simulink library "lib_dGrid"  (R2023b)
settings: Solver=VariableStepAuto  StartTime=0.0  StopTime=10.0  RelTol=1e-3
values from neighbouring files (symbols this model uses):
  C_PM = 10e-3    (= 0.01)    [my_MMC_param.m]
  Cbase = 1/Zbase/wb    (= 3.10849498226e-05)    [my_MMC_param.m]
  f0 = 50/fb    (= 1)    [my_MMC_param.m]
  Fn_filter = 1000    [my_MMC_param.m]
  Fnom = 50    [my_MMC_param.m]
  GFL_APC = 1    [Analysis_Main.m]    (also in initSimu.m; my_MMC_param.m)
  GFL_DVC = 2    [Analysis_Main.m]    (also in initSimu.m; my_MMC_param.m)
  GFM_APC = 3; (values programmed in EMT models)    [Analysis_Main.m]    (also in initSimu.m; my_MMC_param.m = 3)
  GFM_VF = 0    [my_MMC_param.m]
  Ibase = 2*Sbase/(3*Ubase)    [my_MMC_param.m]
  Idcb = Sbase/Udcb    [my_MMC_param.m]
  Ki_Iccsc = 5.15    [my_MMC_param.m]
  Ki_Ireg = CCCTRL.CC.ki    [my_MMC_param.m]
  Ki_Izscc = 100    [my_MMC_param.m]
  Ki_PLL = 1/(CCCTRL.PLL.v0*CCCTRL.PLL.T^2)    [my_MMC_param.m]
  Ki_Preg = 1.0*10    (= 10)    [my_MMC_param.m]
  Ki_Qreg = 1.0*10    (= 10)    [my_MMC_param.m]
  Ki_VAC_GFL = 50    [my_MMC_param.m]
  Ki_VACreg = 10    [my_MMC_param.m]
  Ki_VDCreg = 10    [my_MMC_param.m]
  Ki_WtReg = Kp_WtReg / 0.025    (= 1600)    [my_MMC_param.m]
  Kp_Iccsc = 0.21    [my_MMC_param.m]
  Kp_Ireg = CCCTRL.CC.kp    [my_MMC_param.m]
  Kp_Izscc = 10    [my_MMC_param.m]
  Kp_PLL = 2/CCCTRL.PLL.v0/CCCTRL.PLL.T    [my_MMC_param.m]
  Kp_Preg = 0.5/3*1    (= 0.166666666667)    [my_MMC_param.m]
  Kp_Qreg = 0.5/3*1    (= 0.166666666667)    [my_MMC_param.m]
  Kp_VAC_GFL = 0.5    [my_MMC_param.m]
  Kp_VACreg = 0.01    [my_MMC_param.m]
  Kp_VDCreg = 1    [my_MMC_param.m]
  Kp_WtReg = 40    [my_MMC_param.m]
  Kpv_GFM = 1    [my_MMC_param.m]
  Kpwm = 0.5    [my_MMC_param.m]
  Larm = Larm_pu*(Zbase/wb)    (= 0.0488923985178)    [my_MMC_param.m]
  Lff = Larm_pu/2    (= 0.075)    [my_MMC_param.m]
  Limits_Ireg = [ 2.0  -2.0]    [my_MMC_param.m]
  Limits_Preg = [ 2, -2 ]    [my_MMC_param.m]
  Limits_Qreg = 2*[ 0.42, -0.42 ]    [my_MMC_param.m]
  Limits_VACreg = [ 1.3  -1.3]    [my_MMC_param.m]
  Limits_VDCreg = [ 2.0  -2.0]    [my_MMC_param.m]
  MMC1 = MMC    [Analysis_Main.m]    (also in initSimu.m)
  Nb_PM = 400    [my_MMC_param.m]
  PhaseDelay = 1.0*Ts_Control*2*pi*50    (= 0.0628318530718)    [my_MMC_param.m]
  Pnom = 1000e6    (= 1000000000)    [my_MMC_param.m]
  Rarm = Rarm_pu*Zbase    (= 0.1536)    [my_MMC_param.m]
  Slope_Pref = 0.5    [my_MMC_param.m]
  Slope_Qref = 0.5    [my_MMC_param.m]
  Slope_Vdc_ref = Vnom_dc/2    (= 320000)    [my_MMC_param.m]
  Tdeblock = 1.5    [my_MMC_param.m]
  Ton_CROSSreg = Ton_PQreg+3    (= 7)    [my_MMC_param.m]
  Ton_PQreg = 4    [my_MMC_param.m]
  Ton_VDCreg = 1.5    [my_MMC_param.m]
  Ts = Ts_Control    (= 0.0002)    [my_MMC_param.m]
  Ts_Control = Ts_Power*2    (= 0.0002)    [my_MMC_param.m]
  Ts_Power = 20e-6 * 5    (= 0.0001)    [my_MMC_param.m]
  Ubase = sqrt(2/3)*Vnom_sec    [my_MMC_param.m]
  Udcb = 2*Ubase    [my_MMC_param.m]
  Vc0_PM = 0    [my_MMC_param.m]
  Vnom_dc = 640e3    (= 640000)    [my_MMC_param.m]
  Vnom_sec = 320e3    (= 320000)    [my_MMC_param.m]
  wb = 2*pi*fb    (= 314.159265359)    [my_MMC_param.m]
  Wt_ref_pu = 0.5 * C_PM * (Vnom_dc/Nb_PM)^2 * Nb_PM * 6 / Pnom    (= 0.03072)    [my_MMC_param.m]
undefined symbols (not defined in the file or in its folder): ControlSampleTime, DiscIntNeverNeededParam, MMC, PLL, VSM
libraries: simulink x50, spsCurrentMeasurementLib x20, spsSecondOrderFilterLib x20, spsDiodeLib x12, spsControlledVoltageSourceLib x12, spsSeriesRLCBranchLib x10, spsFirstOrderFilterLib x9, spsVoltageMeasurementLib x8, spsMeanLib x7, FriedrichLibrary x6, $bdroot x6, powerlib_extras x4
(part 1 of 8)
settings Model: Creator=uk081705  LastModifiedBy=uk081705

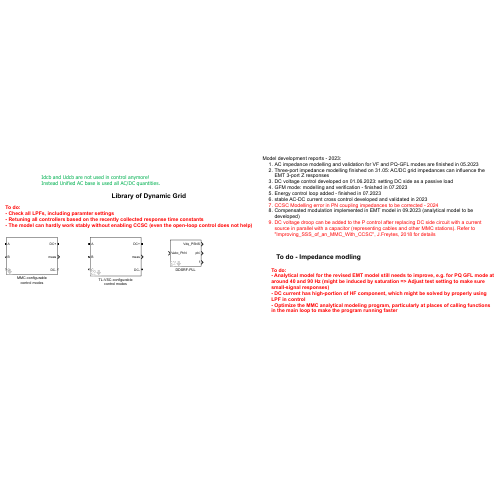
[thumbnail: Simulink's stored preview of the top-level diagram]
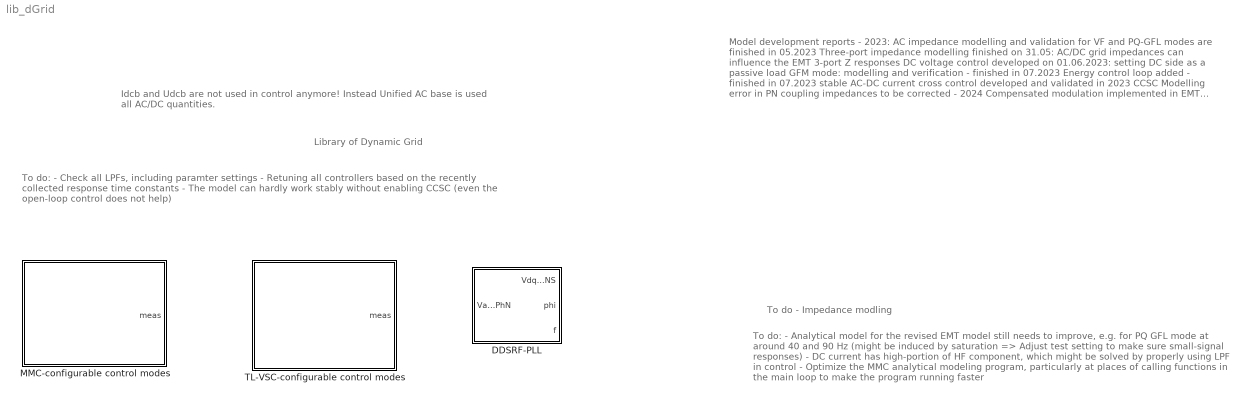
== system lib_dGrid ==
  note: To do:
      | - Check all LPFs, including paramter settings
      | - Retuning all controllers based on the recently collected response time constants
      | - The model can hardly work stably without enabling CCSC (even the open-loop control does not help)
  note: Library of Dynamic Grid
  note: Model development reports - 2023:
      | AC impedance modelling and validation for VF and PQ-GFL modes are finished in 05.2023
      | Three-port impedance modelling finished on 31.05: AC/DC grid impedances can influence the EMT 3-port Z responses
      | DC voltage control developed on 01.06.2023: setting DC side as a passive load
      | GFM mode: modelling and verification - finished in 07.2023
      | Energy control loop added - finished in 07.2023
      | stable AC-DC current cross control developed and validated in 2023
      | CCSC Modelling error in PN coupling impedances to be corrected - 2024
      | Compensated modulation implemented in EMT model in 09.2023 (analytical model to be developed)
      | DC voltage droop can be added to the P control after replacing DC side circuit with a current source in parallel with a capacitor (representing cables and other MMC stations). Refer to "Improving_SSS_of_an_MMC_With_CCSC", J.Freytes, 2018 for details
  note: Idcb and Udcb are not used in control anymore!
      | Instead Unified AC base is used all AC/DC quantities.
  note: To do:
      | - Analytical model for the revised EMT model still needs to improve, e.g. for PQ GFL mode at around 40 and 90 Hz (might be induced by saturation => Adjust test setting to make sure small-signal responses)
      | - DC current has high-portion of HF component, which might be solved by properly using LPF in control
      | - Optimize the MMC analytical modeling program, particularly at places of calling functions in the main loop to make the program running faster
  note: To do - Impedance modling
  DDSRF-PLL : Subsystem  AncestorBlock=FriedrichLibrary/Discrete Stuff/DDSRF-PLL  mask{Kp_PLL=PLL.kp, Ki_PLL=PLL.ki, Kd_PLL=0, Tpt1=0.005, Ts=ControlSampleTime}
      mask prompts: Kp_PLL "Proportional Gain PLL"; Ki_PLL "Integral Gain PLL"; Kd_PLL "Differential Gain PLL"; Tpt1 "PT1 Settling Time"; Ts "SampleTime"
      mask DialogControl DescGroupVar Prompt: DDSRF PLL
      mask DialogControl DescTextVar Prompt: Discrete implementation of a double decoupled sychronous reference frame phase locked loop.
  MMC-configurable control modes : Subsystem  mask{CtrlMode=MMC.CtrlMode, Ctrl=MMC.Ctrl, Set=MMC.Set}
      mask prompts: CtrlMode "GFM-VF0,GFL-APC1,GFL-DVC2, GFM-APC3"; Ctrl "CtrlStru"; Set "SetStru"
      settings: PortSchema="{\"entries\":[{\"content\":{\"sides\":[{\"content\":{\"connectorIds\":[\"LConn1\",\"LConn2\",\"LConn3\"]},\"type\":\"ConnectorPlacement.EquallySpacedRectSide\",\"uuid\":\"c923a6b0-d2fc-4b8e-a4b1-de94c3223959\"},{\"content\":{\"connectorIds\":[\"RConn1\",\"Out1\",\"RConn2\"],\"side\":\"RIGHT\"},\"type\":\"ConnectorPlacement.EquallySpacedRectSide\",\"uuid\":\"6efd3e4a-f3ae-490c-a9d1-2120854778d7\"},{\"content\":{\"side\":\"TOP\"},\"type\":\"ConnectorPlacement.EquallySpacedRectSide\",\"uuid\":\"54cc3c02-aa24-440c-8051-39c65b165fe4\"}]},\"type\":\"ConnectorPlacement.EquallySpacedConnector\",\"uuid\":\"58f4ddb9-74a8-4d52-977f-61a3e301d753\"}],\"packageUris\":[\"http://schema.mathworks.com/mf0/Connector/R2020b\"],\"version\":\"1.0\"}"
      mask DialogControl AAM Prompt: MMC-Averaged Arm Model
  TL-VSC-configurable control modes : Subsystem  AncestorBlock=Library_dynaGrid/MMC - configurable control & operating modes  mask{CtrlMode=MMC1.CtrlMode, Ctrl=MMC1.Ctrl, Set=MMC1.Set}
      mask prompts: CtrlMode "GFM-VF0,GFL-APC1,GFL-DVC2, GFM-APC3"; Ctrl "CtrlStru"; Set "SetStru"
      settings: PortSchema="{\"entries\":[{\"content\":{\"sides\":[{\"content\":{\"connectorIds\":[\"LConn1\",\"LConn2\",\"LConn3\"]},\"type\":\"ConnectorPlacement.EquallySpacedRectSide\",\"uuid\":\"c923a6b0-d2fc-4b8e-a4b1-de94c3223959\"},{\"content\":{\"connectorIds\":[\"RConn1\",\"Out1\",\"RConn2\"],\"side\":\"RIGHT\"},\"type\":\"ConnectorPlacement.EquallySpacedRectSide\",\"uuid\":\"6efd3e4a-f3ae-490c-a9d1-2120854778d7\"},{\"content\":{\"side\":\"TOP\"},\"type\":\"ConnectorPlacement.EquallySpacedRectSide\",\"uuid\":\"54cc3c02-aa24-440c-8051-39c65b165fe4\"}]},\"type\":\"ConnectorPlacement.EquallySpacedConnector\",\"uuid\":\"58f4ddb9-74a8-4d52-977f-61a3e301d753\"}],\"packageUris\":[\"http://schema.mathworks.com/mf0/Connector/R2020b\"],\"version\":\"1.0\"}"
      mask DialogControl AAM Prompt: MMC-Averaged Arm Model

== system lib_dGrid/DDSRF-PLL ==
  Vabc_PhN : Inport
  Angle Integrator [SI] : FriedrichLibrary/Discrete Stuff/Angle Integrator [SI]  Ts=Ts
  Bus Creator : BusCreator  Inputs=2
  Demux1 : Demux  Outputs=2
  PhN->ab0 : FriedrichLibrary/Transformations/PhN->ab0  SystemSampleTime=-1  VariantActivationTime=update diagram  AllowFlexibleInterface=on  Latency=0  AutoFrameSizeCalculation=off
  Selector : Selector  InputPortWidth=3  IndexOptions=Index vector (dialog)  Indices=2  OutputSizes=1
  Selector1 : Selector  InputPortWidth=3  IndexOptions=Index vector (dialog)  Indices=[2 1]  OutputSizes=1
  Trigonometric Function1 : Trigonometry  Operator=atan2
  ab0->dq0 PSNS : FriedrichLibrary/Transformations/ab0->dq0 PSNS  T1=0.0045
  discrete PID : FriedrichLibrary/Discrete Stuff/discrete PID  Kp=Kp_PLL  Ki=Ki_PLL  Kd=Kd_PLL  Ts=Ts  x_init=2*pi*50
  "omega -> f" : Gain  Gain=1/2/pi
  Vdq_PSNS : Outport  VectorParamsAs1DForOutWhenUnconnected=off
  phi : Outport  Port=2  VectorParamsAs1DForOutWhenUnconnected=off
  f : Outport  Port=3  VectorParamsAs1DForOutWhenUnconnected=off
  wires:
  Trigonometric Function1/1 -> Angle Integrator [SI]/2
  PhN->ab0/1 -> Selector1/1, ab0->dq0 PSNS/1
  "omega -> f"/1 -> f/1
  Angle Integrator [SI]/1 -> ab0->dq0 PSNS/2, phi/1
  discrete PID/1 -> "omega -> f"/1, Angle Integrator [SI]/1
  Selector/1 -> discrete PID/1
  ab0->dq0 PSNS/1 -> Selector/1, Bus Creator/1  "PosSeq"
  ab0->dq0 PSNS/2 -> Bus Creator/2  "NegSeq"
  Bus Creator/1 -> Vdq_PSNS/1
  Vabc_PhN/1 -> PhN->ab0/1
  Demux1/2 -> Trigonometric Function1/2
  Selector1/1 -> Demux1/1
  Demux1/1 -> Trigonometric Function1/1

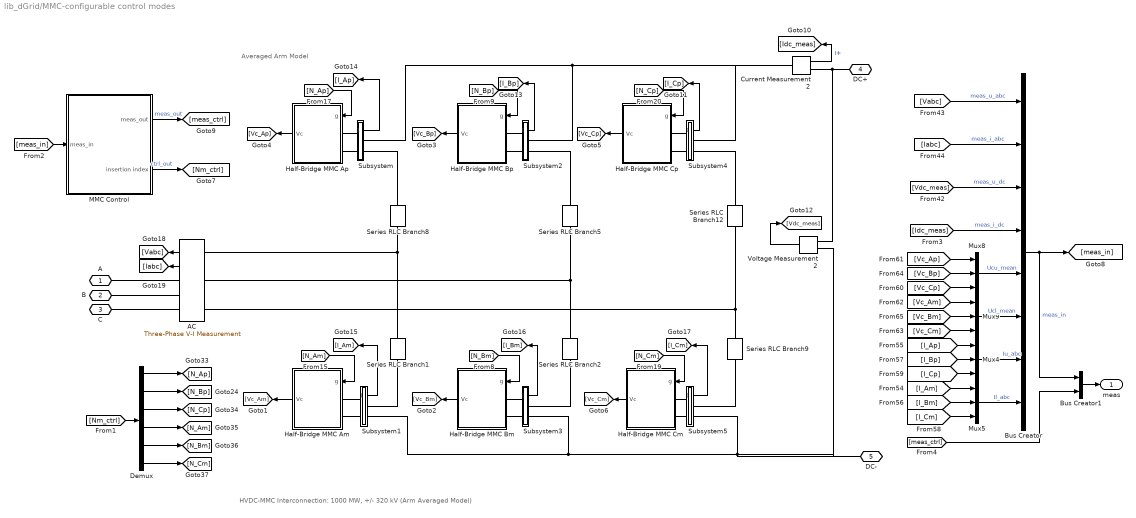
== system lib_dGrid/MMC-configurable control modes ==
  note: HVDC-MMC Interconnection: 1000 MW, +/- 320 kV (Arm Averaged Model)
  note: Averaged Arm Model
  AC : spsThreePhaseVIMeasurementLib/Three-Phase V-I Measurement  VoltageMeasurement=phase-to-ground  SetLabelV=off  LabelV=Vabc  Vpu=off  VpuLL=off  CurrentMeasurement=yes  SetLabelI=off  LabelI=Iabc  Ipu=off  Pbase=Pnom  Vbase=Vnom_ac  OutputType=Complex  PhasorSimulation=off  PSBequivalent=0
      link override Vabc: TagVisibility=local
  Bus Creator : BusCreator  Inputs=8
  Bus Creator1 : BusCreator  Inputs=2
  Current Measurement2 : spsCurrentMeasurementLib/Current Measurement  PhasorSimulation=off  OutputType=Complex  PSBequivalent=0
  Demux : Demux  Outputs=6
  Half-Bridge MMC Am : Subsystem  mask(Half-Bridge MMC - Aggregate Model){n=Nb_PM, C=C_PM, Vc_Initial=Vc0_PM, Ts=Ts_Power}
      mask prompts: n "Number of power modules"; C "Capacitor value (F):"; Vc_Initial "Capacitor initial voltage (V):"; Ts "Sample time (s):"
      mask help:
      | Implement a half-bridge Modular Multilevel Converter (MMC) using a switching-function model where only one equivalent module is used to represent all power modules.
      |
      | The control signal is a two-element vector [ Nin, Nbl ], where Nin represents the number of inserted modules and Nbl represents the number of modules in the blocked-state. The output Vc (capacitor voltage) has only one element and gives the average value of the capacitors modules.
      |
      | With this aggregate model, it is assumed that capacitor voltage of all power modules are well-balanced. However, control system dynamics, converter harmonics content and circulating currents phenomena are all-well represented. The model runs a lot faster than the detailed model which uses two switching devices and one capacitor for each individual power module. This aggregate model is also well-suited for real-time simulation.
      settings: AttributesFormatString=(Aggregate model of %<n> PM)
      mask Display:
      | x1=0.0;
      | plot([0.17 0.5]+x1,[0.93 0.93])
      | plot([0.5 0.5]+x1,[0.93,0.80])
      | plot([0.5 0.38]+x1,[0.80 0.74])
      | plot([0.38 0.38]+x1,[0.80 0.62])
      | plot([0.38 0.5]+x1,[0.68 0.62])
      | plot([0.5 0.5]+x1,[0.62 0.52])
      | plot([0.45 0.5 0.43]+x1,[0.68 0.62 0.60])
      | %
      | y1=0.40-0.03;
      | plot([0.5 0.5]+x1,[0.93,0.80]-y1)
      | plot([0.5 0.38]+x1,[0.80 0.74]-y1)
      | plot([0.38 0.38]+x1,[0.80 0.62]-y1)
      | plot([0.38 0.5]+x1,[0.68 0.62]-y1)
      | plot([0.5 0.5]+x1,[0.62 0.52]-y1)
      | plot([0.45 0.5 0.43]+x1,[0.68 0.62 0.60]-y1)
      | plot([0.5 0.5]+x1,[0.2,0.10])
      | plot([0.17 0.5]+x1,[0.1 0.1])
      | %
      | plot([0.5 0.6]+x1,[0.84 0.84]+0.03)
      | plot([0.6 0.6]+x1,[0.84 0.74]+0.03)
      | plot([0.6 0.56]+x1,[0.74 0.69]+0.03)
      | plot([0.6 0.64]+x1,[0.74 0.69]+0.03)
      | plot([0.56 0.64]+x1,[0.69 0.69]+0.03)
      | plot([0.6 0.6]+x1,[0.69 0.57]+0.03)
      | plot([0.5 0.6]+x1,[0.57 0.57]+0.03)
      | plot([0.55 0.65]+x1,[0.74 0.74]+0.03)
      | %
      | y2=0.4-0.03;
      | plot([0.5 0.6]+x1,[0.84 0.84]-y2)
      | plot([0.6 0.6]+x1,[0.84 0.74]-y2)
      | plot([0.6 0.56]+x1,[0.74 0.69]-y2)
      | plot([0.6 0.64]+x1,[0.74 0.69]-y2)
      | plot([0.56 0.64]+x1,[0.69 0.69]-y2)
      | plot([0.6 0.6]+x1,[0.69 0.57]-y2)
      | plot([0.5 0.6]+x1,[0.57 0.57]-y2)
      | plot([0.55 0.65]+x1,[0.74 0.74]-y2)
      | %
      | plot([0.5 0.75]+x1,[0.53 0.53])
      | plot([0.75 0.75]+x1,[0.53 0.57])
      | plot([0.75 0.75]+x1,[0.61 0.65])
      | plot([0.75 0.75]+x1,[0.69 0.73])
      | plot([0.75 0.75]+x1,[0.77 0.81])
      | plot([0.75 0.75]+x1,[0.09 0.07])
      | plot([0.75 0.75]+x1,[0.04 0.01])
      | %
      | plot([0.34 0.34]+x1,[0.65 0.75])
      | plot([0.28 0.34]+x1,[0.7 0.7])
      | %
      | plot([0.34 0.34]+x1,[0.65 0.75]-y2)
      | plot([0.28 0.34]+x1,[0.7 0.7]-y2)
      | %
      | %Capacitor
      | plot([0.16 0.16],[0.93 0.54])
      | plot([0.16 0.16],[0.47 0.10])
      | plot([0.04 0.27],[0.54 0.54])
      | plot([0.04 0.27],[0.47 0.47])
      | %
      | plot([0.5 0.75],[0.1 0.1])
      | % text(0.78,0.5,'1')
      | % text(0.78,0.12,'2')
      | %
      | color('blue')
      | port_label('input',1,'N')
  Half-Bridge MMC Ap : Subsystem  mask(Half-Bridge MMC - Aggregate Model){n=Nb_PM, C=C_PM, Vc_Initial=Vc0_PM, Ts=Ts_Power}
      mask prompts: n "Number of power modules"; C "Capacitor value (F):"; Vc_Initial "Capacitor initial voltage (V):"; Ts "Sample time (s):"
      mask help:
      | Implement a half-bridge Modular Multilevel Converter (MMC) using a switching-function model where only one equivalent module is used to represent all power modules.
      |
      | The control signal is a two-element vector [ Nin, Nbl ], where Nin represents the number of inserted modules and Nbl represents the number of modules in the blocked-state. The output Vc (capacitor voltage) has only one element and gives the average value of the capacitors modules.
      |
      | With this aggregate model, it is assumed that capacitor voltage of all power modules are well-balanced. However, control system dynamics, converter harmonics content and circulating currents phenomena are all-well represented. The model runs a lot faster than the detailed model which uses two switching devices and one capacitor for each individual power module. This aggregate model is also well-suited for real-time simulation.
      settings: AttributesFormatString=(Aggregate model of %<n> PM)
      mask Display:
      | x1=0.0;
      | plot([0.17 0.5]+x1,[0.93 0.93])
      | plot([0.5 0.5]+x1,[0.93,0.80])
      | plot([0.5 0.38]+x1,[0.80 0.74])
      | plot([0.38 0.38]+x1,[0.80 0.62])
      | plot([0.38 0.5]+x1,[0.68 0.62])
      | plot([0.5 0.5]+x1,[0.62 0.52])
      | plot([0.45 0.5 0.43]+x1,[0.68 0.62 0.60])
      | %
      | y1=0.40-0.03;
      | plot([0.5 0.5]+x1,[0.93,0.80]-y1)
      | plot([0.5 0.38]+x1,[0.80 0.74]-y1)
      | plot([0.38 0.38]+x1,[0.80 0.62]-y1)
      | plot([0.38 0.5]+x1,[0.68 0.62]-y1)
      | plot([0.5 0.5]+x1,[0.62 0.52]-y1)
      | plot([0.45 0.5 0.43]+x1,[0.68 0.62 0.60]-y1)
      | plot([0.5 0.5]+x1,[0.2,0.10])
      | plot([0.17 0.5]+x1,[0.1 0.1])
      | %
      | plot([0.5 0.6]+x1,[0.84 0.84]+0.03)
      | plot([0.6 0.6]+x1,[0.84 0.74]+0.03)
      | plot([0.6 0.56]+x1,[0.74 0.69]+0.03)
      | plot([0.6 0.64]+x1,[0.74 0.69]+0.03)
      | plot([0.56 0.64]+x1,[0.69 0.69]+0.03)
      | plot([0.6 0.6]+x1,[0.69 0.57]+0.03)
      | plot([0.5 0.6]+x1,[0.57 0.57]+0.03)
      | plot([0.55 0.65]+x1,[0.74 0.74]+0.03)
      | %
      | y2=0.4-0.03;
      | plot([0.5 0.6]+x1,[0.84 0.84]-y2)
      | plot([0.6 0.6]+x1,[0.84 0.74]-y2)
      | plot([0.6 0.56]+x1,[0.74 0.69]-y2)
      | plot([0.6 0.64]+x1,[0.74 0.69]-y2)
      | plot([0.56 0.64]+x1,[0.69 0.69]-y2)
      | plot([0.6 0.6]+x1,[0.69 0.57]-y2)
      | plot([0.5 0.6]+x1,[0.57 0.57]-y2)
      | plot([0.55 0.65]+x1,[0.74 0.74]-y2)
      | %
      | plot([0.5 0.75]+x1,[0.53 0.53])
      | plot([0.75 0.75]+x1,[0.53 0.57])
      | plot([0.75 0.75]+x1,[0.61 0.65])
      | plot([0.75 0.75]+x1,[0.69 0.73])
      | plot([0.75 0.75]+x1,[0.77 0.81])
      | plot([0.75 0.75]+x1,[0.09 0.07])
      | plot([0.75 0.75]+x1,[0.04 0.01])
      | %
      | plot([0.34 0.34]+x1,[0.65 0.75])
      | plot([0.28 0.34]+x1,[0.7 0.7])
      | %
      | plot([0.34 0.34]+x1,[0.65 0.75]-y2)
      | plot([0.28 0.34]+x1,[0.7 0.7]-y2)
      | %
      | %Capacitor
      | plot([0.16 0.16],[0.93 0.54])
      | plot([0.16 0.16],[0.47 0.10])
      | plot([0.04 0.27],[0.54 0.54])
      | plot([0.04 0.27],[0.47 0.47])
      | %
      | plot([0.5 0.75],[0.1 0.1])
      | % text(0.78,0.5,'1')
      | % text(0.78,0.12,'2')
      | %
      | color('blue')
      | port_label('input',1,'N')
  Half-Bridge MMC Bm : Subsystem  mask(Half-Bridge MMC - Aggregate Model){n=Nb_PM, C=C_PM, Vc_Initial=Vc0_PM, Ts=Ts_Power}
      mask prompts: n "Number of power modules"; C "Capacitor value (F):"; Vc_Initial "Capacitor initial voltage (V):"; Ts "Sample time (s):"
      mask help:
      | Implement a half-bridge Modular Multilevel Converter (MMC) using a switching-function model where only one equivalent module is used to represent all power modules.
      |
      | The control signal is a two-element vector [ Nin, Nbl ], where Nin represents the number of inserted modules and Nbl represents the number of modules in the blocked-state. The output Vc (capacitor voltage) has only one element and gives the average value of the capacitors modules.
      |
      | With this aggregate model, it is assumed that capacitor voltage of all power modules are well-balanced. However, control system dynamics, converter harmonics content and circulating currents phenomena are all-well represented. The model runs a lot faster than the detailed model which uses two switching devices and one capacitor for each individual power module. This aggregate model is also well-suited for real-time simulation.
      settings: AttributesFormatString=(Aggregate model of %<n> PM)
      mask Display:
      | x1=0.0;
      | plot([0.17 0.5]+x1,[0.93 0.93])
      | plot([0.5 0.5]+x1,[0.93,0.80])
      | plot([0.5 0.38]+x1,[0.80 0.74])
      | plot([0.38 0.38]+x1,[0.80 0.62])
      | plot([0.38 0.5]+x1,[0.68 0.62])
      | plot([0.5 0.5]+x1,[0.62 0.52])
      | plot([0.45 0.5 0.43]+x1,[0.68 0.62 0.60])
      | %
      | y1=0.40-0.03;
      | plot([0.5 0.5]+x1,[0.93,0.80]-y1)
      | plot([0.5 0.38]+x1,[0.80 0.74]-y1)
      | plot([0.38 0.38]+x1,[0.80 0.62]-y1)
      | plot([0.38 0.5]+x1,[0.68 0.62]-y1)
      | plot([0.5 0.5]+x1,[0.62 0.52]-y1)
      | plot([0.45 0.5 0.43]+x1,[0.68 0.62 0.60]-y1)
      | plot([0.5 0.5]+x1,[0.2,0.10])
      | plot([0.17 0.5]+x1,[0.1 0.1])
      | %
      | plot([0.5 0.6]+x1,[0.84 0.84]+0.03)
      | plot([0.6 0.6]+x1,[0.84 0.74]+0.03)
      | plot([0.6 0.56]+x1,[0.74 0.69]+0.03)
      | plot([0.6 0.64]+x1,[0.74 0.69]+0.03)
      | plot([0.56 0.64]+x1,[0.69 0.69]+0.03)
      | plot([0.6 0.6]+x1,[0.69 0.57]+0.03)
      | plot([0.5 0.6]+x1,[0.57 0.57]+0.03)
      | plot([0.55 0.65]+x1,[0.74 0.74]+0.03)
      | %
      | y2=0.4-0.03;
      | plot([0.5 0.6]+x1,[0.84 0.84]-y2)
      | plot([0.6 0.6]+x1,[0.84 0.74]-y2)
      | plot([0.6 0.56]+x1,[0.74 0.69]-y2)
      | plot([0.6 0.64]+x1,[0.74 0.69]-y2)
      | plot([0.56 0.64]+x1,[0.69 0.69]-y2)
      | plot([0.6 0.6]+x1,[0.69 0.57]-y2)
      | plot([0.5 0.6]+x1,[0.57 0.57]-y2)
      | plot([0.55 0.65]+x1,[0.74 0.74]-y2)
      | %
      | plot([0.5 0.75]+x1,[0.53 0.53])
      | plot([0.75 0.75]+x1,[0.53 0.57])
      | plot([0.75 0.75]+x1,[0.61 0.65])
      | plot([0.75 0.75]+x1,[0.69 0.73])
      | plot([0.75 0.75]+x1,[0.77 0.81])
      | plot([0.75 0.75]+x1,[0.09 0.07])
      | plot([0.75 0.75]+x1,[0.04 0.01])
      | %
      | plot([0.34 0.34]+x1,[0.65 0.75])
      | plot([0.28 0.34]+x1,[0.7 0.7])
      | %
      | plot([0.34 0.34]+x1,[0.65 0.75]-y2)
      | plot([0.28 0.34]+x1,[0.7 0.7]-y2)
      | %
      | %Capacitor
      | plot([0.16 0.16],[0.93 0.54])
      | plot([0.16 0.16],[0.47 0.10])
      | plot([0.04 0.27],[0.54 0.54])
      | plot([0.04 0.27],[0.47 0.47])
      | %
      | plot([0.5 0.75],[0.1 0.1])
      | % text(0.78,0.5,'1')
      | % text(0.78,0.12,'2')
      | %
      | color('blue')
      | port_label('input',1,'N')
  Half-Bridge MMC Bp : Subsystem  mask(Half-Bridge MMC - Aggregate Model){n=Nb_PM, C=C_PM, Vc_Initial=Vc0_PM, Ts=Ts_Power}
      mask prompts: n "Number of power modules"; C "Capacitor value (F):"; Vc_Initial "Capacitor initial voltage (V):"; Ts "Sample time (s):"
      mask help:
      | Implement a half-bridge Modular Multilevel Converter (MMC) using a switching-function model where only one equivalent module is used to represent all power modules.
      |
      | The control signal is a two-element vector [ Nin, Nbl ], where Nin represents the number of inserted modules and Nbl represents the number of modules in the blocked-state. The output Vc (capacitor voltage) has only one element and gives the average value of the capacitors modules.
      |
      | With this aggregate model, it is assumed that capacitor voltage of all power modules are well-balanced. However, control system dynamics, converter harmonics content and circulating currents phenomena are all-well represented. The model runs a lot faster than the detailed model which uses two switching devices and one capacitor for each individual power module. This aggregate model is also well-suited for real-time simulation.
      settings: AttributesFormatString=(Aggregate model of %<n> PM)
      mask Display:
      | x1=0.0;
      | plot([0.17 0.5]+x1,[0.93 0.93])
      | plot([0.5 0.5]+x1,[0.93,0.80])
      | plot([0.5 0.38]+x1,[0.80 0.74])
      | plot([0.38 0.38]+x1,[0.80 0.62])
      | plot([0.38 0.5]+x1,[0.68 0.62])
      | plot([0.5 0.5]+x1,[0.62 0.52])
      | plot([0.45 0.5 0.43]+x1,[0.68 0.62 0.60])
      | %
      | y1=0.40-0.03;
      | plot([0.5 0.5]+x1,[0.93,0.80]-y1)
      | plot([0.5 0.38]+x1,[0.80 0.74]-y1)
      | plot([0.38 0.38]+x1,[0.80 0.62]-y1)
      | plot([0.38 0.5]+x1,[0.68 0.62]-y1)
      | plot([0.5 0.5]+x1,[0.62 0.52]-y1)
      | plot([0.45 0.5 0.43]+x1,[0.68 0.62 0.60]-y1)
      | plot([0.5 0.5]+x1,[0.2,0.10])
      | plot([0.17 0.5]+x1,[0.1 0.1])
      | %
      | plot([0.5 0.6]+x1,[0.84 0.84]+0.03)
      | plot([0.6 0.6]+x1,[0.84 0.74]+0.03)
      | plot([0.6 0.56]+x1,[0.74 0.69]+0.03)
      | plot([0.6 0.64]+x1,[0.74 0.69]+0.03)
      | plot([0.56 0.64]+x1,[0.69 0.69]+0.03)
      | plot([0.6 0.6]+x1,[0.69 0.57]+0.03)
      | plot([0.5 0.6]+x1,[0.57 0.57]+0.03)
      | plot([0.55 0.65]+x1,[0.74 0.74]+0.03)
      | %
      | y2=0.4-0.03;
      | plot([0.5 0.6]+x1,[0.84 0.84]-y2)
      | plot([0.6 0.6]+x1,[0.84 0.74]-y2)
      | plot([0.6 0.56]+x1,[0.74 0.69]-y2)
      | plot([0.6 0.64]+x1,[0.74 0.69]-y2)
      | plot([0.56 0.64]+x1,[0.69 0.69]-y2)
      | plot([0.6 0.6]+x1,[0.69 0.57]-y2)
      | plot([0.5 0.6]+x1,[0.57 0.57]-y2)
      | plot([0.55 0.65]+x1,[0.74 0.74]-y2)
      | %
      | plot([0.5 0.75]+x1,[0.53 0.53])
      | plot([0.75 0.75]+x1,[0.53 0.57])
      | plot([0.75 0.75]+x1,[0.61 0.65])
      | plot([0.75 0.75]+x1,[0.69 0.73])
      | plot([0.75 0.75]+x1,[0.77 0.81])
      | plot([0.75 0.75]+x1,[0.09 0.07])
      | plot([0.75 0.75]+x1,[0.04 0.01])
      | %
      | plot([0.34 0.34]+x1,[0.65 0.75])
      | plot([0.28 0.34]+x1,[0.7 0.7])
      | %
      | plot([0.34 0.34]+x1,[0.65 0.75]-y2)
      | plot([0.28 0.34]+x1,[0.7 0.7]-y2)
      | %
      | %Capacitor
      | plot([0.16 0.16],[0.93 0.54])
      | plot([0.16 0.16],[0.47 0.10])
      | plot([0.04 0.27],[0.54 0.54])
      | plot([0.04 0.27],[0.47 0.47])
      | %
      | plot([0.5 0.75],[0.1 0.1])
      | % text(0.78,0.5,'1')
      | % text(0.78,0.12,'2')
      | %
      | color('blue')
      | port_label('input',1,'N')
  Half-Bridge MMC Cm : Subsystem  mask(Half-Bridge MMC - Aggregate Model){n=Nb_PM, C=C_PM, Vc_Initial=Vc0_PM, Ts=Ts_Power}
      mask prompts: n "Number of power modules"; C "Capacitor value (F):"; Vc_Initial "Capacitor initial voltage (V):"; Ts "Sample time (s):"
      mask help:
      | Implement a half-bridge Modular Multilevel Converter (MMC) using a switching-function model where only one equivalent module is used to represent all power modules.
      |
      | The control signal is a two-element vector [ Nin, Nbl ], where Nin represents the number of inserted modules and Nbl represents the number of modules in the blocked-state. The output Vc (capacitor voltage) has only one element and gives the average value of the capacitors modules.
      |
      | With this aggregate model, it is assumed that capacitor voltage of all power modules are well-balanced. However, control system dynamics, converter harmonics content and circulating currents phenomena are all-well represented. The model runs a lot faster than the detailed model which uses two switching devices and one capacitor for each individual power module. This aggregate model is also well-suited for real-time simulation.
      settings: AttributesFormatString=(Aggregate model of %<n> PM)
      mask Display:
      | x1=0.0;
      | plot([0.17 0.5]+x1,[0.93 0.93])
      | plot([0.5 0.5]+x1,[0.93,0.80])
      | plot([0.5 0.38]+x1,[0.80 0.74])
      | plot([0.38 0.38]+x1,[0.80 0.62])
      | plot([0.38 0.5]+x1,[0.68 0.62])
      | plot([0.5 0.5]+x1,[0.62 0.52])
      | plot([0.45 0.5 0.43]+x1,[0.68 0.62 0.60])
      | %
      | y1=0.40-0.03;
      | plot([0.5 0.5]+x1,[0.93,0.80]-y1)
      | plot([0.5 0.38]+x1,[0.80 0.74]-y1)
      | plot([0.38 0.38]+x1,[0.80 0.62]-y1)
      | plot([0.38 0.5]+x1,[0.68 0.62]-y1)
      | plot([0.5 0.5]+x1,[0.62 0.52]-y1)
      | plot([0.45 0.5 0.43]+x1,[0.68 0.62 0.60]-y1)
      | plot([0.5 0.5]+x1,[0.2,0.10])
      | plot([0.17 0.5]+x1,[0.1 0.1])
      | %
      | plot([0.5 0.6]+x1,[0.84 0.84]+0.03)
      | plot([0.6 0.6]+x1,[0.84 0.74]+0.03)
      | plot([0.6 0.56]+x1,[0.74 0.69]+0.03)
      | plot([0.6 0.64]+x1,[0.74 0.69]+0.03)
      | plot([0.56 0.64]+x1,[0.69 0.69]+0.03)
      | plot([0.6 0.6]+x1,[0.69 0.57]+0.03)
      | plot([0.5 0.6]+x1,[0.57 0.57]+0.03)
      | plot([0.55 0.65]+x1,[0.74 0.74]+0.03)
      | %
      | y2=0.4-0.03;
      | plot([0.5 0.6]+x1,[0.84 0.84]-y2)
      | plot([0.6 0.6]+x1,[0.84 0.74]-y2)
      | plot([0.6 0.56]+x1,[0.74 0.69]-y2)
      | plot([0.6 0.64]+x1,[0.74 0.69]-y2)
      | plot([0.56 0.64]+x1,[0.69 0.69]-y2)
      | plot([0.6 0.6]+x1,[0.69 0.57]-y2)
      | plot([0.5 0.6]+x1,[0.57 0.57]-y2)
      | plot([0.55 0.65]+x1,[0.74 0.74]-y2)
      | %
      | plot([0.5 0.75]+x1,[0.53 0.53])
      | plot([0.75 0.75]+x1,[0.53 0.57])
      | plot([0.75 0.75]+x1,[0.61 0.65])
      | plot([0.75 0.75]+x1,[0.69 0.73])
      | plot([0.75 0.75]+x1,[0.77 0.81])
      | plot([0.75 0.75]+x1,[0.09 0.07])
      | plot([0.75 0.75]+x1,[0.04 0.01])
      | %
      | plot([0.34 0.34]+x1,[0.65 0.75])
      | plot([0.28 0.34]+x1,[0.7 0.7])
      | %
      | plot([0.34 0.34]+x1,[0.65 0.75]-y2)
      | plot([0.28 0.34]+x1,[0.7 0.7]-y2)
      | %
      | %Capacitor
      | plot([0.16 0.16],[0.93 0.54])
      | plot([0.16 0.16],[0.47 0.10])
      | plot([0.04 0.27],[0.54 0.54])
      | plot([0.04 0.27],[0.47 0.47])
      | %
      | plot([0.5 0.75],[0.1 0.1])
      | % text(0.78,0.5,'1')
      | % text(0.78,0.12,'2')
      | %
      | color('blue')
      | port_label('input',1,'N')
  Half-Bridge MMC Cp : Subsystem  mask(Half-Bridge MMC - Aggregate Model){n=Nb_PM, C=C_PM, Vc_Initial=Vc0_PM, Ts=Ts_Power}
      mask prompts: n "Number of power modules"; C "Capacitor value (F):"; Vc_Initial "Capacitor initial voltage (V):"; Ts "Sample time (s):"
      mask help:
      | Implement a half-bridge Modular Multilevel Converter (MMC) using a switching-function model where only one equivalent module is used to represent all power modules.
      |
      | The control signal is a two-element vector [ Nin, Nbl ], where Nin represents the number of inserted modules and Nbl represents the number of modules in the blocked-state. The output Vc (capacitor voltage) has only one element and gives the average value of the capacitors modules.
      |
      | With this aggregate model, it is assumed that capacitor voltage of all power modules are well-balanced. However, control system dynamics, converter harmonics content and circulating currents phenomena are all-well represented. The model runs a lot faster than the detailed model which uses two switching devices and one capacitor for each individual power module. This aggregate model is also well-suited for real-time simulation.
      settings: AttributesFormatString=(Aggregate model of %<n> PM)
      mask Display:
      | x1=0.0;
      | plot([0.17 0.5]+x1,[0.93 0.93])
      | plot([0.5 0.5]+x1,[0.93,0.80])
      | plot([0.5 0.38]+x1,[0.80 0.74])
      | plot([0.38 0.38]+x1,[0.80 0.62])
      | plot([0.38 0.5]+x1,[0.68 0.62])
      | plot([0.5 0.5]+x1,[0.62 0.52])
      | plot([0.45 0.5 0.43]+x1,[0.68 0.62 0.60])
      | %
      | y1=0.40-0.03;
      | plot([0.5 0.5]+x1,[0.93,0.80]-y1)
      | plot([0.5 0.38]+x1,[0.80 0.74]-y1)
      | plot([0.38 0.38]+x1,[0.80 0.62]-y1)
      | plot([0.38 0.5]+x1,[0.68 0.62]-y1)
      | plot([0.5 0.5]+x1,[0.62 0.52]-y1)
      | plot([0.45 0.5 0.43]+x1,[0.68 0.62 0.60]-y1)
      | plot([0.5 0.5]+x1,[0.2,0.10])
      | plot([0.17 0.5]+x1,[0.1 0.1])
      | %
      | plot([0.5 0.6]+x1,[0.84 0.84]+0.03)
      | plot([0.6 0.6]+x1,[0.84 0.74]+0.03)
      | plot([0.6 0.56]+x1,[0.74 0.69]+0.03)
      | plot([0.6 0.64]+x1,[0.74 0.69]+0.03)
      | plot([0.56 0.64]+x1,[0.69 0.69]+0.03)
      | plot([0.6 0.6]+x1,[0.69 0.57]+0.03)
      | plot([0.5 0.6]+x1,[0.57 0.57]+0.03)
      | plot([0.55 0.65]+x1,[0.74 0.74]+0.03)
      | %
      | y2=0.4-0.03;
      | plot([0.5 0.6]+x1,[0.84 0.84]-y2)
      | plot([0.6 0.6]+x1,[0.84 0.74]-y2)
      | plot([0.6 0.56]+x1,[0.74 0.69]-y2)
      | plot([0.6 0.64]+x1,[0.74 0.69]-y2)
      | plot([0.56 0.64]+x1,[0.69 0.69]-y2)
      | plot([0.6 0.6]+x1,[0.69 0.57]-y2)
      | plot([0.5 0.6]+x1,[0.57 0.57]-y2)
      | plot([0.55 0.65]+x1,[0.74 0.74]-y2)
      | %
      | plot([0.5 0.75]+x1,[0.53 0.53])
      | plot([0.75 0.75]+x1,[0.53 0.57])
      | plot([0.75 0.75]+x1,[0.61 0.65])
      | plot([0.75 0.75]+x1,[0.69 0.73])
      | plot([0.75 0.75]+x1,[0.77 0.81])
      | plot([0.75 0.75]+x1,[0.09 0.07])
      | plot([0.75 0.75]+x1,[0.04 0.01])
      | %
      | plot([0.34 0.34]+x1,[0.65 0.75])
      | plot([0.28 0.34]+x1,[0.7 0.7])
      | %
      | plot([0.34 0.34]+x1,[0.65 0.75]-y2)
      | plot([0.28 0.34]+x1,[0.7 0.7]-y2)
      | %
      | %Capacitor
      | plot([0.16 0.16],[0.93 0.54])
      | plot([0.16 0.16],[0.47 0.10])
      | plot([0.04 0.27],[0.54 0.54])
      | plot([0.04 0.27],[0.47 0.47])
      | %
      | plot([0.5 0.75],[0.1 0.1])
      | % text(0.78,0.5,'1')
      | % text(0.78,0.12,'2')
      | %
      | color('blue')
      | port_label('input',1,'N')
  MMC Control : Subsystem
      mask Display: disp('Controllers')
  Mux{4..5,8..9} (4 alike) : Mux  Inputs=3
  Series RLC Branch{1..2,5,8..9,12} (6 alike) : spsSeriesRLCBranchLib/Series RLC Branch  LConnTagsString=__new0  RConnTagsString=__new0  BranchType=RL  Resistance=Rarm  Inductance=Larm  SetiL0=off  InitialCurrent=0  Capacitance=1e-6  Setx0=off  InitialVoltage=0  Measurements=None
  Subsystem : Subsystem
  Subsystem1 : Subsystem
  Subsystem2 : Subsystem
  Subsystem3 : Subsystem
  Subsystem4 : Subsystem
  Subsystem5 : Subsystem
  Voltage Measurement2 : spsVoltageMeasurementLib/Voltage Measurement  PhasorSimulation=off  OutputType=Complex  PSBequivalent=0
  A : PMIOPort  Side=Left
  B : PMIOPort  Port=2  Side=Left
  C : PMIOPort  Port=3  Side=Left
  DC+ : PMIOPort  Port=4  Side=Right
  DC- : PMIOPort  Port=5  Side=Right
  meas : Outport  VectorParamsAs1DForOutWhenUnconnected=off
  wires:
  [N_Bp] -> Half-Bridge MMC Bp/1(g)
  Half-Bridge MMC Bm/1(Vc) -> [Vc_Bm]
  Half-Bridge MMC Ap/1(Vc) -> [Vc_Ap]
  [N_Bm] -> Half-Bridge MMC Bm/1(g)
  Half-Bridge MMC Bp/1(Vc) -> [Vc_Bp]
  [N_Cm] -> Half-Bridge MMC Cm/1(g)
  Half-Bridge MMC Cp/1(Vc) -> [Vc_Cp]
  [N_Am] -> Half-Bridge MMC Am/1(g)
  [N_Ap] -> Half-Bridge MMC Ap/1(g)
  Half-Bridge MMC Cm/1(Vc) -> [Vc_Cm]
  [N_Cp] -> Half-Bridge MMC Cp/1(g)
  Half-Bridge MMC Am/1(Vc) -> [Vc_Am]
  [Vc_Cm] -> Mux9/3
  [Vc_Bm] -> Mux9/2
  [Vc_Ap] -> Mux8/1
  [I_Cp] -> Mux4/3
  [Vc_Bp] -> Mux8/2
  [Vc_Cp] -> Mux8/3
  [I_Bp] -> Mux4/2
  [Vc_Am] -> Mux9/1
  [I_Cm] -> Mux5/3
  [I_Am] -> Mux5/1
  [I_Ap] -> Mux4/1
  [I_Bm] -> Mux5/2
  Current Measurement2/1 -> [Idc_meas]  "I+"
  Voltage Measurement2/1 -> [Vdc_meas]
  [Vabc] -> Bus Creator/1  "meas_u_abc"
  [Iabc] -> Bus Creator/2  "meas_i_abc"
  [Vdc_meas] -> Bus Creator/3  "meas_u_dc"
  Mux8/1 -> Bus Creator/5  "Ucu_mean"
  Mux9/1 -> Bus Creator/6  "Ucl_mean"
  [Idc_meas] -> Bus Creator/4  "meas_i_dc"
  Demux/1 -> [N_Ap]
  Demux/2 -> [N_Bp]
  Demux/3 -> [N_Cp]
  Demux/5 -> [N_Bm]
  Demux/6 -> [N_Cm]
  Bus Creator1/1 -> meas/1
  Bus Creator/1 -> [meas_in], Bus Creator1/1  "meas_in"
  Subsystem4/1(I_Cp) -> [I_Cp]
  Subsystem2/1(I_Bp) -> [I_Bp]
  Subsystem/1(I_Ap) -> [I_Ap]
  Subsystem5/1(I_Cm) -> [I_Cm]
  Subsystem3/1(I_Bm) -> [I_Bm]
  Subsystem1/1(I_Am) -> [I_Am]
  Demux/4 -> [N_Am]
  [Nm_ctrl] -> Demux/1
  AC/1 -> [Vabc]
  AC/2 -> [Iabc]
  [meas_in] -> MMC Control/1(meas_in)
  MMC Control/1(meas_out) -> [meas_ctrl]  "meas_out"
  MMC Control/2(insertion index) -> [Nm_ctrl]  "ctrl_out"
  [meas_ctrl] -> Bus Creator1/2
  Mux4/1 -> Bus Creator/7  "Iu_abc"
  Mux5/1 -> Bus Creator/8  "Il_abc"
  connections:
  Series RLC Branch9/RConn1 -- Subsystem5/RConn1
  Half-Bridge MMC Cp/LConn1 -- Subsystem4/LConn1
  Subsystem3/RConn2 -- Subsystem1/RConn2 -- Voltage Measurement2/LConn2 -- DC-/RConn1 -- Subsystem5/RConn2
  Half-Bridge MMC Am/LConn2 -- Subsystem1/LConn2
  Subsystem2/RConn1 -- Subsystem4/RConn1 -- Current Measurement2/LConn1 -- Subsystem/RConn1
  Half-Bridge MMC Bm/LConn1 -- Subsystem3/LConn1
  Series RLC Branch8/RConn1 -- Series RLC Branch1/LConn1 -- AC/LConn1
  Subsystem4/RConn2 -- Series RLC Branch12/LConn1
  Half-Bridge MMC Bp/LConn2 -- Subsystem2/LConn2
  Subsystem2/RConn2 -- Series RLC Branch5/LConn1
  Half-Bridge MMC Bp/LConn1 -- Subsystem2/LConn1
  Half-Bridge MMC Am/LConn1 -- Subsystem1/LConn1
  Series RLC Branch2/RConn1 -- Subsystem3/RConn1
  Half-Bridge MMC Cm/LConn2 -- Subsystem5/LConn2
  Series RLC Branch12/RConn1 -- Series RLC Branch9/LConn1 -- AC/LConn3
  Subsystem/RConn2 -- Series RLC Branch8/LConn1
  Half-Bridge MMC Ap/LConn1 -- Subsystem/LConn1
  Series RLC Branch1/RConn1 -- Subsystem1/RConn1
  Half-Bridge MMC Ap/LConn2 -- Subsystem/LConn2
  Half-Bridge MMC Bm/LConn2 -- Subsystem3/LConn2
  Half-Bridge MMC Cm/LConn1 -- Subsystem5/LConn1
  Half-Bridge MMC Cp/LConn2 -- Subsystem4/LConn2
  Series RLC Branch5/RConn1 -- Series RLC Branch2/LConn1 -- AC/LConn2
  B/RConn1 -- AC/RConn2
  C/RConn1 -- AC/RConn3
  A/RConn1 -- AC/RConn1
  Current Measurement2/RConn1 -- Voltage Measurement2/LConn1 -- DC+/RConn1

== system lib_dGrid/TL-VSC-configurable control modes ==
  note: TL-VSC HVDC Interconnection: 1000 MW, +/- 320 kV
  note: DC Capacitor
  note: Smoothing reactor
  note: Adapt the Capacitance parameter based on the aggrevated C of all C_PMs in MMC
  AC : spsThreePhaseVIMeasurementLib/Three-Phase V-I Measurement  VoltageMeasurement=phase-to-ground  SetLabelV=off  LabelV=Vabc  Vpu=off  VpuLL=off  CurrentMeasurement=yes  SetLabelI=off  LabelI=Iabc  Ipu=off  Pbase=Pnom  Vbase=Vnom_ac  OutputType=Complex  PhasorSimulation=off  PSBequivalent=0
      link override Vabc: TagVisibility=local
  Bconv : spsThreePhaseVIMeasurementLib/Three-Phase V-I Measurement  VoltageMeasurement=phase-to-ground  SetLabelV=on  LabelV=Uc_abc  Vpu=on  VpuLL=off  CurrentMeasurement=yes  SetLabelI=on  LabelI=Ic_abc  Ipu=on  Pbase=1000e6  Vbase=320e3  OutputType=Complex  PhasorSimulation=off  PSBequivalent=0
  Bus Creator : BusCreator  Inputs=4
  Bus Creator1 : BusCreator  Inputs=2
  Cn1 : spsSeriesRLCBranchLib/Series RLC Branch  LConnTagsString=__new0  RConnTagsString=__new0  BranchType=C  Resistance=[]  Inductance=[]  SetiL0=off  InitialCurrent=0  Capacitance=70e-6  Setx0=off  InitialVoltage=0  Measurements=None
  Cp1 : spsSeriesRLCBranchLib/Series RLC Branch  LConnTagsString=__new0  RConnTagsString=__new0  BranchType=C  Resistance=[]  Inductance=[]  SetiL0=off  InitialCurrent=0  Capacitance=70e-6  Setx0=off  InitialVoltage=0  Measurements=None
  Current Measurement2 : spsCurrentMeasurementLib/Current Measurement  PhasorSimulation=off  OutputType=Complex  PSBequivalent=0
  Filters 60Hz2 : Subsystem
      mask Display: disp('AC filters\n200 Mvar')
  Ground : spsGroundLib/Ground  LConnTagsString=a
  Ln1 : spsSeriesRLCBranchLib/Series RLC Branch  Commented=through  LConnTagsString=__new0  RConnTagsString=__new0  BranchType=RL  Resistance=0.0251  Inductance=8.0e-3  SetiL0=off  InitialCurrent=0  Capacitance=[]  Setx0=off  InitialVoltage=0  Measurements=Branch current
  Lp1 : spsSeriesRLCBranchLib/Series RLC Branch  Commented=through  LConnTagsString=__new0  RConnTagsString=__new0  BranchType=RL  Resistance=0.0251  Inductance=8.0e-3  SetiL0=off  InitialCurrent=0  Capacitance=[]  Setx0=off  InitialVoltage=0  Measurements=Branch current
  Phase reactor 0.15 p.u. : spsThreePhaseSeriesRLCBranchLib/Three-Phase Series RLC Branch  LConnTagsString=A|B|C  RConnTagsString=A|B|C  BranchType=RL  Resistance=0.0015*(320^2 / 1000)  Inductance=0.15* (320^2 / 1000) / (2*pi*Fnom)  Capacitance=1.0  Measurements=None
  Two-Level Converter : spsTwoLevelConverterLib/Two-Level Converter  ModelType=Switching devices  Ron=1e-3  Rs=1e6  Cs=inf  Vforward=[0,0]  Ron_Diode=1e-3  Rs_Diode=1e6  Cs_Diode=inf  Vf_Diode=1e-3  Rs_CurrentSource=inf  Ron_ACsource=1e-3
      settings: LibrarySourceBlock=sps_lib/Power Electronics/Two-Level Converter
  VSC Control : Subsystem
      mask Display: disp('Controllers')
  Voltage Measurement2 : spsVoltageMeasurementLib/Voltage Measurement  PhasorSimulation=off  OutputType=Complex  PSBequivalent=0
  A : PMIOPort  Side=Left
  B : PMIOPort  Port=2  Side=Left
  C : PMIOPort  Port=3  Side=Left
  DC+ : PMIOPort  Port=4  Side=Right
  DC- : PMIOPort  Port=5  Side=Right
  meas : Outport  VectorParamsAs1DForOutWhenUnconnected=off
  wires:
  Current Measurement2/1 -> [Idc_meas]  "I+"
  [Vabc] -> Bus Creator/1  "meas_u_abc"
  [Iabc] -> Bus Creator/2  "meas_i_abc"
  [Vdc_meas] -> Bus Creator/3  "meas_u_dc"
  [Idc_meas] -> Bus Creator/4  "meas_i_dc"
  Bus Creator1/1 -> meas/1
  Bus Creator/1 -> Bus Creator1/1, [meas_in]  "meas_in"
  AC/1 -> [Vabc]
  AC/2 -> [Iabc]
  [meas_in] -> VSC Control/1(meas_in)
  VSC Control/1(meas_out) -> [meas_ctrl]  "meas_out"
  VSC Control/2(modulation index) -> [Pulses]  "ctrl_out"
  [meas_ctrl] -> Bus Creator1/2
  Voltage Measurement2/1 -> [Vdc_meas]
  [Pulses] -> Two-Level Converter/1
  [Block] -> Two-Level Converter/2
  VSC Control/3(BlkSig) -> [Block]
  connections:
  DC-/RConn1 -- Ln1/RConn1 -- Voltage Measurement2/LConn2
  B/RConn1 -- AC/RConn2
  C/RConn1 -- AC/RConn3
  A/RConn1 -- AC/RConn1
  Current Measurement2/RConn1 -- Voltage Measurement2/LConn1 -- DC+/RConn1
  Cn1/RConn1 -- Ln1/LConn1 -- Two-Level Converter/RConn2
  Filters 60Hz2/LConn3 -- Phase reactor 0.15 p.u./LConn3 -- AC/LConn3
  Cp1/RConn1 -- Ground/LConn1 -- Cn1/LConn1
  Cp1/LConn1 -- Two-Level Converter/RConn1 -- Lp1/LConn1
  Filters 60Hz2/LConn2 -- Phase reactor 0.15 p.u./LConn2 -- AC/LConn2
  Phase reactor 0.15 p.u./RConn1 -- Bconv/LConn1
  Two-Level Converter/LConn1 -- Bconv/RConn1
  Two-Level Converter/LConn3 -- Bconv/RConn3
  Two-Level Converter/LConn2 -- Bconv/RConn2
  Phase reactor 0.15 p.u./RConn3 -- Bconv/LConn3
  Phase reactor 0.15 p.u./RConn2 -- Bconv/LConn2
  Lp1/RConn1 -- Current Measurement2/LConn1
  Phase reactor 0.15 p.u./LConn1 -- Filters 60Hz2/LConn1 -- AC/LConn1

== system lib_dGrid/MMC-configurable control modes/Half-Bridge MMC Am ==
  g : Inport
  HalfBridgeMMC_Agt_Discrete : Subsystem  mask{n=n, C=C, Vc_Initial=Vc_Initial, Ron_Diode=1e-3, Rs_Diode=1e6, Cs_Diode=inf, Vf_Diode=0}
      mask prompts: n "Number of bridges:"; C "Capacitor value (F):"; Vc_Initial "Initial capacitor voltage (V):"; Ron_Diode "Diode on-state resistance (Ohms)"; Rs_Diode "Diode snubber resistance (Ohms)"; Cs_Diode "Diode snubber capacitance (F)"; Vf_Diode "Diode forward voltage (V)"
  1 : PMIOPort  Side=Left
  2 : PMIOPort  Port=2  Side=Left
  Vc : Outport  VectorParamsAs1DForOutWhenUnconnected=off
  wires:
  HalfBridgeMMC_Agt_Discrete/1(Vc) -> Vc/1
  g/1 -> HalfBridgeMMC_Agt_Discrete/1(N)
  connections:
  1/RConn1 -- HalfBridgeMMC_Agt_Discrete/LConn1
  2/RConn1 -- HalfBridgeMMC_Agt_Discrete/LConn2

== system lib_dGrid/MMC-configurable control modes/Half-Bridge MMC Ap ==
  g : Inport
  HalfBridgeMMC_Agt_Discrete : Subsystem  mask{n=n, C=C, Vc_Initial=Vc_Initial, Ron_Diode=1e-3, Rs_Diode=1e6, Cs_Diode=inf, Vf_Diode=0}
      mask prompts: n "Number of bridges:"; C "Capacitor value (F):"; Vc_Initial "Initial capacitor voltage (V):"; Ron_Diode "Diode on-state resistance (Ohms)"; Rs_Diode "Diode snubber resistance (Ohms)"; Cs_Diode "Diode snubber capacitance (F)"; Vf_Diode "Diode forward voltage (V)"
  1 : PMIOPort  Side=Left
  2 : PMIOPort  Port=2  Side=Left
  Vc : Outport  VectorParamsAs1DForOutWhenUnconnected=off
  wires:
  g/1 -> HalfBridgeMMC_Agt_Discrete/1(N)
  HalfBridgeMMC_Agt_Discrete/1(Vc) -> Vc/1
  connections:
  2/RConn1 -- HalfBridgeMMC_Agt_Discrete/LConn2
  1/RConn1 -- HalfBridgeMMC_Agt_Discrete/LConn1

== system lib_dGrid/MMC-configurable control modes/Half-Bridge MMC Bm ==
  g : Inport
  HalfBridgeMMC_Agt_Discrete : Subsystem  mask{n=n, C=C, Vc_Initial=Vc_Initial, Ron_Diode=1e-3, Rs_Diode=1e6, Cs_Diode=inf, Vf_Diode=0}
      mask prompts: n "Number of bridges:"; C "Capacitor value (F):"; Vc_Initial "Initial capacitor voltage (V):"; Ron_Diode "Diode on-state resistance (Ohms)"; Rs_Diode "Diode snubber resistance (Ohms)"; Cs_Diode "Diode snubber capacitance (F)"; Vf_Diode "Diode forward voltage (V)"
  1 : PMIOPort  Side=Left
  2 : PMIOPort  Port=2  Side=Left
  Vc : Outport  VectorParamsAs1DForOutWhenUnconnected=off
  wires:
  g/1 -> HalfBridgeMMC_Agt_Discrete/1(N)
  HalfBridgeMMC_Agt_Discrete/1(Vc) -> Vc/1
  connections:
  2/RConn1 -- HalfBridgeMMC_Agt_Discrete/LConn2
  1/RConn1 -- HalfBridgeMMC_Agt_Discrete/LConn1

== system lib_dGrid/MMC-configurable control modes/Half-Bridge MMC Bp ==
  g : Inport
  HalfBridgeMMC_Agt_Discrete : Subsystem  mask{n=n, C=C, Vc_Initial=Vc_Initial, Ron_Diode=1e-3, Rs_Diode=1e6, Cs_Diode=inf, Vf_Diode=0}
      mask prompts: n "Number of bridges:"; C "Capacitor value (F):"; Vc_Initial "Initial capacitor voltage (V):"; Ron_Diode "Diode on-state resistance (Ohms)"; Rs_Diode "Diode snubber resistance (Ohms)"; Cs_Diode "Diode snubber capacitance (F)"; Vf_Diode "Diode forward voltage (V)"
  1 : PMIOPort  Side=Left
  2 : PMIOPort  Port=2  Side=Left
  Vc : Outport  VectorParamsAs1DForOutWhenUnconnected=off
  wires:
  HalfBridgeMMC_Agt_Discrete/1(Vc) -> Vc/1
  g/1 -> HalfBridgeMMC_Agt_Discrete/1(N)
  connections:
  1/RConn1 -- HalfBridgeMMC_Agt_Discrete/LConn1
  2/RConn1 -- HalfBridgeMMC_Agt_Discrete/LConn2

== system lib_dGrid/MMC-configurable control modes/Half-Bridge MMC Cm ==
  g : Inport
  HalfBridgeMMC_Agt_Discrete : Subsystem  mask{n=n, C=C, Vc_Initial=Vc_Initial, Ron_Diode=1e-3, Rs_Diode=1e6, Cs_Diode=inf, Vf_Diode=0}
      mask prompts: n "Number of bridges:"; C "Capacitor value (F):"; Vc_Initial "Initial capacitor voltage (V):"; Ron_Diode "Diode on-state resistance (Ohms)"; Rs_Diode "Diode snubber resistance (Ohms)"; Cs_Diode "Diode snubber capacitance (F)"; Vf_Diode "Diode forward voltage (V)"
  1 : PMIOPort  Side=Left
  2 : PMIOPort  Port=2  Side=Left
  Vc : Outport  VectorParamsAs1DForOutWhenUnconnected=off
  wires:
  HalfBridgeMMC_Agt_Discrete/1(Vc) -> Vc/1
  g/1 -> HalfBridgeMMC_Agt_Discrete/1(N)
  connections:
  1/RConn1 -- HalfBridgeMMC_Agt_Discrete/LConn1
  2/RConn1 -- HalfBridgeMMC_Agt_Discrete/LConn2

== system lib_dGrid/MMC-configurable control modes/Half-Bridge MMC Cp ==
  g : Inport
  HalfBridgeMMC_Agt_Discrete : Subsystem  mask{n=n, C=C, Vc_Initial=Vc_Initial, Ron_Diode=1e-3, Rs_Diode=1e6, Cs_Diode=inf, Vf_Diode=0}
      mask prompts: n "Number of bridges:"; C "Capacitor value (F):"; Vc_Initial "Initial capacitor voltage (V):"; Ron_Diode "Diode on-state resistance (Ohms)"; Rs_Diode "Diode snubber resistance (Ohms)"; Cs_Diode "Diode snubber capacitance (F)"; Vf_Diode "Diode forward voltage (V)"
  1 : PMIOPort  Side=Left
  2 : PMIOPort  Port=2  Side=Left
  Vc : Outport  VectorParamsAs1DForOutWhenUnconnected=off
  wires:
  g/1 -> HalfBridgeMMC_Agt_Discrete/1(N)
  HalfBridgeMMC_Agt_Discrete/1(Vc) -> Vc/1
  connections:
  2/RConn1 -- HalfBridgeMMC_Agt_Discrete/LConn2
  1/RConn1 -- HalfBridgeMMC_Agt_Discrete/LConn1
